simulink model "sim_1_twolink_joint_control_ideal"  (R2021a)
settings: Solver=ode15s  StartTime=0.0  StopTime=15  RelTol=1e-5  EnableMultiTasking=on
values from neighbouring files (symbols this model uses):
  b1 = 0.01    [sim_params.m]    (also in sim_params_force.m)
  b2 = 0.01    [sim_params.m]    (also in sim_params_force.m)
  D = [zeros(n); eye(n)]    [control_comparison_script.m]    (also in gen_twolink_ss.m = reshape([0.0,0.0,0.0,0.0,0.0,0.0,0.0,0.0],[4,2]))
  D_T_Q = D'*Q    [control_comparison_script.m]
  epsilon = 0.1    [control_comparison_script.m]
  g = 9.80665    [sim_params.m]    (also in sim_params_force.m)
  Kd1 = 2.5    [control_comparison_script.m]
  Kd1_grav = 2.5    [control_comparison_script.m]
  Kd1_inv = 12    [control_comparison_script.m]
  Kd1_robust = 7    [control_comparison_script.m]
  Kd2 = 0.5    [control_comparison_script.m]
  Kd2_grav = 0.5    [control_comparison_script.m]
  Kd2_inv = 15    [control_comparison_script.m]
  Kd2_robust = 35    [control_comparison_script.m]
  Klqr = lqr(A,B,Q,R)    [control_comparison_script.m]
  Kp1 = 30    [control_comparison_script.m]
  Kp1_grav = 15    [control_comparison_script.m]
  Kp1_inv = 25    [control_comparison_script.m]
  Kp1_robust = 25    [control_comparison_script.m]
  Kp2 = 7    [control_comparison_script.m]
  Kp2_grav = 3.5    [control_comparison_script.m]
  Kp2_inv = 50    [control_comparison_script.m]
  Kp2_robust = 45    [control_comparison_script.m]
  Kpp = place(A,B,p)    [control_comparison_script.m]
  L1x = 0.3    [sim_params.m]    (also in sim_params_force.m)
  L1y = 0.050    (= 0.05)    [sim_params.m]    (also in sim_params_force.m)
  L1z = 0.05    [sim_params.m]    (also in sim_params_force.m)
  L2x = 0.15    [sim_params.m]    (also in sim_params_force.m = 0.3)
  L2y = 0.05    [sim_params.m]    (also in sim_params_force.m)
  L2z = 0.05    [sim_params.m]    (also in sim_params_force.m)
  m1 = m1*1.25    [control_comparison_script.m]    (also in sim_params.m = 2.775; sim_params_force.m = 2.775)
  m2 = m2*1.25    [control_comparison_script.m]    (also in sim_params.m = 1.3875; sim_params_force.m = 2.775)
  N1 = 100    [control_comparison_script.m]
  N1_grav = 100    [control_comparison_script.m]
  N1_inv = 50    [control_comparison_script.m]
  N1_robust = 50    [control_comparison_script.m]
  N2 = 100    [control_comparison_script.m]
  N2_grav = 100    [control_comparison_script.m]
  N2_inv = 50    [control_comparison_script.m]
  N2_robust = 50    [control_comparison_script.m]
  rho = [1;1]    [control_comparison_script.m]
  theta1_0 = 0    [sim_params.m]    (also in sim_params_force.m = 1.57079632679)
  theta1_dot_0 = 0    [sim_params.m]    (also in sim_params_force.m)
  theta2_0 = 0    [sim_params.m]    (also in sim_params_force.m = -1.57079632679)
  theta2_dot_0 = 0    [sim_params.m]    (also in sim_params_force.m)
  Tsample = 0.001    [sim_params.m]    (also in sim_params_force.m)
undefined symbols (not defined in the file or in its folder): Kd, Ki, Kp, N, sigbuilder_block, X, Y, Z
libraries: pid_lib x12, sm_lib x11, nesl_utility x10, simulink_extras x8, spsFirstOrderFilterLib x4, dspmtrx3 x1
(part 1 of 3)
settings Model: Creator=bhorton  LastModifiedBy=Petronas-Tareq
settings SolverCC: ZeroCrossAlgorithm=Adaptive  AlgebraicLoopSolver=TrustRegion
settings DataIOCC: ReturnWorkspaceOutputs=off
settings OptimizationCC: LifeSpan=inf
settings DebuggingCC: SFUnexpectedBacktrackingDiag=warning  SFNoUnconditionalDefaultTransitionDiag=warning  SFExecutionAtInitializationDiag=none  SFMachineParentedDataDiag=warning  ArithmeticOperatorsInVariantConditions=warning
settings SFSimCC: SimUseLocalCustomCode=off  CustomCodeUndefinedFunction=UseInterfaceOnly
settings RTWCC: RTWUseLocalCustomCode=off
settings CodeAppCC: StateflowObjectComments=on
settings GRTTargetCC: TargetLangStandard=C89/C90 (ANSI)
settings ConfigComp: CovMetricSettings=dw  CovSaveCumulativeToWorkspaceVar=on  CovSaveSingleToWorkspaceVar=on  CovExternalEMLEnable=off
settings SimscapeCC: SimscapeNormalizeSystem=off  SimscapeLogType=all  SimscapeLogDataHistory=10000
settings ExplorerConfigSet: InternalSimMechanicsExplorerSettings="<ExplorerConfiguration><canonicalview>planar_xy</canonicalview><AnimationSetting><BasePlaybackSpeed>1.0</BasePlaybackSpeed><PlaybackSpeedFactor>4.0</PlaybackSpeedFactor></AnimationSetting><TilePanel><TileInfo><Tiles Columns=\"1\" Count=\"1\" Rows=\"1\"><Column Weight=\"1\"/><Row Weight=\"1\"/><Tile Height=\"1\" Width=\"1\" X=\"0\" Y=\"0\"/></Tiles></TileInfo><SceneInfo><SceneViewer><BGColor><R>0</R><G>0</G><B>0</B></BGColor><Camera><DoPerspective>off</DoPerspective><Position><X>0.0447898824465682299</X><Y>-0.016656403258507535</Y><Z>0.999999954328562035</Z></Position><Center><X>0.0447898824465682299</X><Y>-0.016656403258507535</Y><Z>-4.56714379648559543e-08</Z></Center><Up><X>0</X><Y>1</Y><Z>0</Z></Up><ViewLimDist>1</ViewLimDist><YLim>0.67213509984740738</YLim><XLim>1.22520332234454554</XLim></Camera></SceneViewer></SceneInfo></TilePanel><MechEditorPanel><Cameras/><GfxPanelCameraMap/><VideoCreator><PlaybackSpeedRatio>1</PlaybackSpeedRatio><FrameRate>30</FrameRate><VideoFormat>Motion JPEG AVI</VideoFormat><FrameSize>auto</FrameSize></VideoCreator></MechEditorPanel></ExplorerConfiguration>"

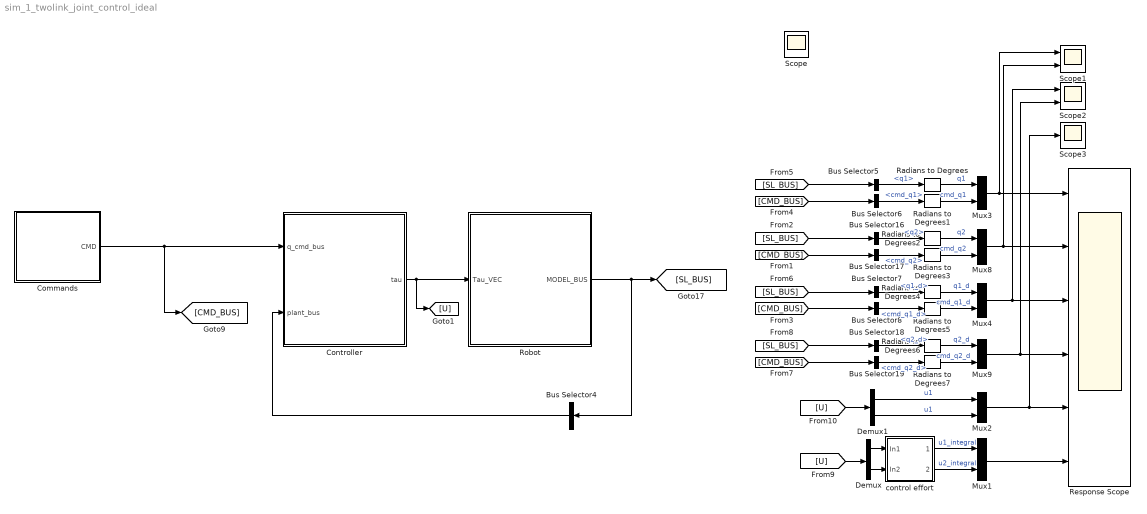
== system sim_1_twolink_joint_control_ideal ==
  Bus Selector16 : BusSelector  OutputSignals=q2
  Bus Selector17 : BusSelector  OutputSignals=cmd_q2
  Bus Selector18 : BusSelector  OutputSignals=q2_d
  Bus Selector19 : BusSelector  OutputSignals=cmd_q2_d
  Bus Selector4 : BusSelector  OutputSignals=q1_dd,q2_dd,q1_d,q2_d,q1,q2  OutputAsBus=on
  Bus Selector5 : BusSelector  OutputSignals=q1
  Bus Selector6 : BusSelector  OutputSignals=cmd_q1
  Bus Selector7 : BusSelector  OutputSignals=q1_d
  Bus Selector8 : BusSelector  OutputSignals=cmd_q1_d
  Commands : Subsystem  Variant=on  VariantControlMode=label  LabelModeActiveChoice=step
  Controller : Subsystem  Variant=on  VariantControlMode=label  LabelModeActiveChoice=LQR_control  PropagateVariantConditions=on
  Demux : Demux  Outputs=2
  Demux1 : Demux  Outputs=2
  Mux{1..4,8..9} (6 alike) : Mux  Inputs=2
  Radians to Degrees{,1..7} (8 alike) : simulink_extras/Transformations/Radians to Degrees
  Response Scope : Scope  NumInputPorts=6
  Robot : Subsystem  Variant=on  VariantControlMode=label  LabelModeActiveChoice=Choice
  Scope1 : Scope  NumInputPorts=2
  Scope2 : Scope  NumInputPorts=2
  Scope3 : Scope
  control effort : Subsystem
  Scope : Scope
  wires:
  Bus Selector4/1 -> Controller/2(plant_bus)
  Controller/1(tau) -> Robot/1(Tau_VEC), [U]
  Commands/1(CMD) -> [CMD_BUS], Controller/1(q_cmd_bus)
  Robot/1(MODEL_BUS) -> [SL_BUS], Bus Selector4/1
  Mux4/1 -> Scope2/1, Response Scope/3
  Mux8/1 -> Scope1/2, Response Scope/2
  Radians to Degrees4/1 -> Mux4/1  "q1_d"
  Radians to Degrees3/1 -> Mux8/2  "cmd_q2"
  Mux3/1 -> Scope1/1, Response Scope/1
  Radians to Degrees6/1 -> Mux9/1  "q2_d"
  Mux9/1 -> Scope2/2, Response Scope/4
  Radians to Degrees5/1 -> Mux4/2  "cmd_q1_d"
  Demux1/1 -> Mux2/1  "u1"
  [SL_BUS] -> Bus Selector7/1
  Bus Selector8/1 -> Radians to Degrees5/1  "<cmd_q1_d>"
  [CMD_BUS] -> Bus Selector8/1
  [U] -> Demux1/1
  Demux1/2 -> Mux2/2  "u1"
  control effort/2(u2_effort) -> Mux1/2  "u2_integral"
  Bus Selector16/1 -> Radians to Degrees2/1  "<q2>"
  [SL_BUS] -> Bus Selector5/1
  Demux/2 -> control effort/2(In2)
  control effort/1(u1_effort) -> Mux1/1  "u1_integral"
  Mux2/1 -> Scope3/1, Response Scope/5
  Bus Selector19/1 -> Radians to Degrees7/1  "<cmd_q2_d>"
  [CMD_BUS] -> Bus Selector19/1
  Bus Selector6/1 -> Radians to Degrees1/1  "<cmd_q1>"
  [SL_BUS] -> Bus Selector16/1
  Bus Selector17/1 -> Radians to Degrees3/1  "<cmd_q2>"
  [SL_BUS] -> Bus Selector18/1
  Radians to Degrees/1 -> Mux3/1  "q1"
  Radians to Degrees2/1 -> Mux8/1  "q2"
  Demux/1 -> control effort/1(In1)
  Bus Selector18/1 -> Radians to Degrees6/1  "<q2_d>"
  Bus Selector7/1 -> Radians to Degrees4/1  "<q1_d>"
  Bus Selector5/1 -> Radians to Degrees/1  "<q1>"
  Radians to Degrees1/1 -> Mux3/2  "cmd_q1"
  [U] -> Demux/1
  Mux1/1 -> Response Scope/6
  [CMD_BUS] -> Bus Selector17/1
  Radians to Degrees7/1 -> Mux9/2  "cmd_q2_d"
  [CMD_BUS] -> Bus Selector6/1

== system sim_1_twolink_joint_control_ideal/Commands ==
  Sinewave command : Subsystem  VariantControl=sinwave
  Step command : Subsystem  VariantControl=step
  Trapezoidal velocity : Subsystem  VariantControl=Trapezoidal velocity
  CMD : Outport

== system sim_1_twolink_joint_control_ideal/Controller ==
  note: 1) Add Subsystem or Model blocks as valid variant choices.
      | 2) You cannot connect blocks at this level. At simulation, connectivity is automatically
      | determined, based on the active variant and port name matching.
  q_cmd_bus : Inport
  plant_bus : Inport  Port=2
  "  LQR Control" : Subsystem  VariantControl=LQR_control
  " Pole Placement Control" : Subsystem  VariantControl=PolePlacement_control
  "Inverse Dynamics control " : Subsystem  VariantControl=Inverse_dynamics_control
  LQR+D Control : Subsystem  VariantControl=LQR_D_control
  PD Control : Subsystem  VariantControl=PD_control
  PD-feedforward-gravity Control : Subsystem  VariantControl=PD_plus_gravity_plus_feadforward
  "PD-gravity Control " : Subsystem  VariantControl=PD_plus_gravity
  PID Control : Subsystem  VariantControl=PID_control
  Pole Placement+D Control : Subsystem  VariantControl=PolePlacement_D_control
  "Robust control " : Subsystem  VariantControl=robust_control
  tau : Outport

== system sim_1_twolink_joint_control_ideal/Robot ==
  note: 1) Add Subsystem or Model blocks as valid variant choices.
      | 2) You cannot connect blocks at this level. At simulation, connectivity is automatically
      | determined, based on the active variant and port name matching.
  Tau_VEC : Inport
  SIMSCAPE_MODEL : Subsystem  VariantControl=Choice_1
  SIMULINK_MODEL : Subsystem  VariantControl=Choice
  MODEL_BUS : Outport

== system sim_1_twolink_joint_control_ideal/control effort ==
  In1 : Inport
  In2 : Inport  Port=2
  Integrator : Integrator
  Integrator1 : Integrator
  Square : Math  Operator=square  SaturateOnIntegerOverflow=on
  Square1 : Math  Operator=square  SaturateOnIntegerOverflow=on
  u1_effort : Outport
  u2_effort : Outport  Port=2
  wires:
  Square/1 -> Integrator/1
  Integrator1/1 -> u2_effort/1  "u2_effort"
  Integrator/1 -> u1_effort/1  "u1_effort"
  Square1/1 -> Integrator1/1
  In2/1 -> Square1/1
  In1/1 -> Square/1

== system sim_1_twolink_joint_control_ideal/Commands/Sinewave command ==
  note: Note: Using derivative blocks without limiters can result in spikes in the signal. Better to manually create the derivative of the signal
  Bus Creator : BusCreator  Inputs=6
  Derivative : Derivative
  Derivative1 : Derivative
  Gain : Gain  Gain=-1
  Gain1 : Gain  Gain=-1
  Sine Wave Function : Sin  SampleTime=0
  Sine Wave Function1 : Sin  Amplitude=0.5  SampleTime=0
  CMD : Outport
  wires:
  Bus Creator/1 -> CMD/1
  Sine Wave Function1/1 -> Gain1/1, Derivative1/1, Bus Creator/6  "cmd_q2"
  Gain1/1 -> Bus Creator/2  "cmd_q2_dd"
  Gain/1 -> Bus Creator/1  "cmd_q1_dd"
  Sine Wave Function/1 -> Gain/1, Derivative/1, Bus Creator/5  "cmd_q1"
  Derivative/1 -> Bus Creator/3  "cmd_q1_d"
  Derivative1/1 -> Bus Creator/4  "cmd_q2_d"

== system sim_1_twolink_joint_control_ideal/Commands/Step command ==
  Bus Creator : BusCreator  Inputs=6
  Constant : Constant  Value=0
  Constant1 : Constant  Value=0
  Derivative : Derivative
  Derivative1 : Derivative
  First-Order Filter : spsFirstOrderFilterLib/First-Order Filter  FilterType=Lowpass  Tc=0.3  Ts=0  Initialize=on  Vac_Init=[0, 0, 100]  Vdc_Init=0  PlotResponse=off  FreqRange="[0,  200,  1]"
  First-Order Filter1 : spsFirstOrderFilterLib/First-Order Filter  FilterType=Lowpass  Tc=0.3  Ts=0  Initialize=on  Vac_Init=[0, 0, 100]  Vdc_Init=0  PlotResponse=off  FreqRange="[0,  200,  1]"
  First-Order Filter2 : spsFirstOrderFilterLib/First-Order Filter  FilterType=Lowpass  Tc=0.2  Ts=0  Initialize=on  Vac_Init=[0, 0, 100]  Vdc_Init=0  PlotResponse=off  FreqRange="[0,  200,  1]"
  First-Order Filter3 : spsFirstOrderFilterLib/First-Order Filter  FilterType=Lowpass  Tc=0.2  Ts=0  Initialize=on  Vac_Init=[0, 0, 100]  Vdc_Init=0  PlotResponse=off  FreqRange="[0,  200,  1]"
  Joint commands : Subsystem  Tag=STV Subsys  LoadFcn=sigbuilder_block('load');  StartFcn=sigbuilder_block('start');  StopFcn=sigbuilder_block('stop');  ClipboardFcn=sigbuilder_block('clipboard');  mask(Sigbuilder block){tuvar=[0:10]}
      mask help: Simulink:masks:SigbuilderBlock_MD
      mask init:
      | if ~strcmp(get_param(bdroot(gcbh),'SimulationStatus'),'stopped') tuvar = sigbuilder_block('maskInit'); end
      settings: CopyFcn=sigbuilder_block('copy');  DeleteFcn=sigbuilder_block('delete');  ModelCloseFcn=sigbuilder_block('modelClose');  PreSaveFcn=sigbuilder_block('preSave');  PauseFcn=sigbuilder_block('pause');  ContinueFcn=sigbuilder_block('continue');  NameChangeFcn=sigbuilder_block('namechange');  OpenFcn=sigbuilder_block('open',[0 36 1152 560.4 ]);  CloseFcn=sigbuilder_block('close');
      mask Display: plot(0, 0, 100, 100,[2, 2, 32, 32, 2], [68, 8, 8, 68, 68],[32, 2], [38, 38], [32, 19, 2],[53, 60, 44], [32, 17, 17, 2],[16, 16, 31, 31]);txt = getActiveGroup(gcbh);text(2, 100, txt,'verticalAlignment', 'top');
  Scope : Scope
  Scope1 : Scope
  Zero-Order Hold : ZeroOrderHold  SampleTime=0.001
  CMD : Outport
  wires:
  Derivative1/1 -> First-Order Filter2/1
  First-Order Filter1/1 -> Bus Creator/5, Derivative/1  "cmd_q1"
  Bus Creator/1 -> Zero-Order Hold/1
  First-Order Filter/1 -> Derivative1/1, Bus Creator/6  "cmd_q2"
  Joint commands/2(cmd_q2) -> First-Order Filter/1  "cmd_q2"
  Derivative/1 -> Scope/1, First-Order Filter3/1
  Joint commands/1(cmd_q1) -> First-Order Filter1/1  "cmd_q1"
  Constant/1 -> Bus Creator/1  "cmd_q1_dd"
  Constant1/1 -> Bus Creator/2  "cmd_q2_dd"
  First-Order Filter2/1 -> Bus Creator/4  "cmd_q2_d"
  First-Order Filter3/1 -> Bus Creator/3  "cmd_q1_d"
  Zero-Order Hold/1 -> Scope1/1, CMD/1

== system sim_1_twolink_joint_control_ideal/Commands/Trapezoidal velocity ==
  Bus Creator : BusCreator  Inputs=6
  Derivative : Derivative
  Derivative2 : Derivative
  Integrator : Integrator
  Integrator1 : Integrator
  Joint commands : Subsystem  Tag=STV Subsys  LoadFcn=sigbuilder_block('load');  StartFcn=sigbuilder_block('start');  StopFcn=sigbuilder_block('stop');  ClipboardFcn=sigbuilder_block('clipboard');  mask(Sigbuilder block){tuvar=[0:10]}
      mask help: Simulink:masks:SigbuilderBlock_MD
      mask init:
      | if ~strcmp(get_param(bdroot(gcbh),'SimulationStatus'),'stopped') tuvar = sigbuilder_block('maskInit'); end
      settings: CopyFcn=sigbuilder_block('copy');  DeleteFcn=sigbuilder_block('delete');  ModelCloseFcn=sigbuilder_block('modelClose');  PreSaveFcn=sigbuilder_block('preSave');  PauseFcn=sigbuilder_block('pause');  ContinueFcn=sigbuilder_block('continue');  NameChangeFcn=sigbuilder_block('namechange');  OpenFcn=sigbuilder_block('open',[4.8 36 1142.4 525.6 ]);  CloseFcn=sigbuilder_block('close');
      mask Display: plot(0, 0, 100, 100,[2, 2, 32, 32, 2], [68, 8, 8, 68, 68],[32, 2], [38, 38], [32, 19, 2],[53, 60, 44], [32, 17, 17, 2],[16, 16, 31, 31]);txt = getActiveGroup(gcbh);text(2, 100, txt,'verticalAlignment', 'top');
  Mux : Mux  Inputs=2
  Scope : Scope
  CMD : Outport
  wires:
  Bus Creator/1 -> CMD/1
  Integrator/1 -> Mux/2, Bus Creator/6  "cmd_q2"
  Derivative2/1 -> Bus Creator/2  "cmd_q2_dd"
  Joint commands/1(cmd_q1_dot) -> Integrator1/1, Derivative/1, Bus Creator/3  "cmd_q1_d"
  Derivative/1 -> Bus Creator/1  "cmd_q1_dd"
  Joint commands/2(cmd_q2_dot) -> Integrator/1, Derivative2/1, Bus Creator/4  "cmd_q2_d"
  Integrator1/1 -> Mux/1, Bus Creator/5  "cmd_q1"
  Mux/1 -> Scope/1

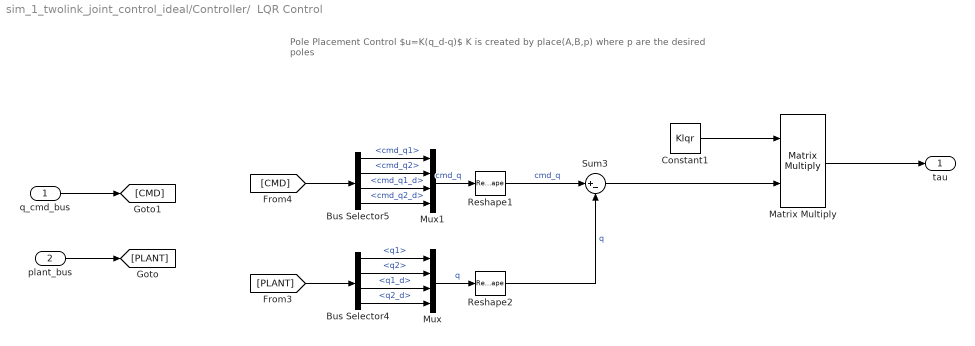
== system sim_1_twolink_joint_control_ideal/Controller/  LQR Control ==
  note: Pole Placement Control
      | $u=K(q_d-q)$
      | K is created by place(A,B,p) where p are the desired poles
  q_cmd_bus : Inport
  plant_bus : Inport  Port=2
  Bus Selector4 : BusSelector  OutputSignals=q1,q2,q1_d,q2_d
  Bus Selector5 : BusSelector  OutputSignals=cmd_q1,cmd_q2,cmd_q1_d,cmd_q2_d
  Constant1 : Constant  Value=Klqr  VectorParams1D=off
  Matrix Multiply : Product  Multiplication=Matrix(*)
  Mux : Mux
  Mux1 : Mux
  Reshape1 : Reshape  OutputDimensionality=Column vector (2-D)
  Reshape2 : Reshape  OutputDimensionality=Column vector (2-D)
  Sum3 : Sum  Inputs=|+-
  tau : Outport
  wires:
  plant_bus/1 -> [PLANT]
  q_cmd_bus/1 -> [CMD]
  [PLANT] -> Bus Selector4/1
  Bus Selector4/3 -> Mux/3  "<q1_d>"
  Bus Selector4/4 -> Mux/4  "<q2_d>"
  Mux/1 -> Reshape2/1  "q"
  Mux1/1 -> Reshape1/1  "cmd_q"
  [CMD] -> Bus Selector5/1
  Bus Selector5/3 -> Mux1/3  "<cmd_q1_d>"
  Bus Selector5/4 -> Mux1/4  "<cmd_q2_d>"
  Bus Selector5/2 -> Mux1/2  "<cmd_q2>"
  Bus Selector5/1 -> Mux1/1  "<cmd_q1>"
  Sum3/1 -> Matrix Multiply/2
  Reshape2/1 -> Sum3/2  "q"
  Reshape1/1 -> Sum3/1  "cmd_q"
  Constant1/1 -> Matrix Multiply/1
  Bus Selector4/1 -> Mux/1  "<q1>"
  Bus Selector4/2 -> Mux/2  "<q2>"
  Matrix Multiply/1 -> tau/1

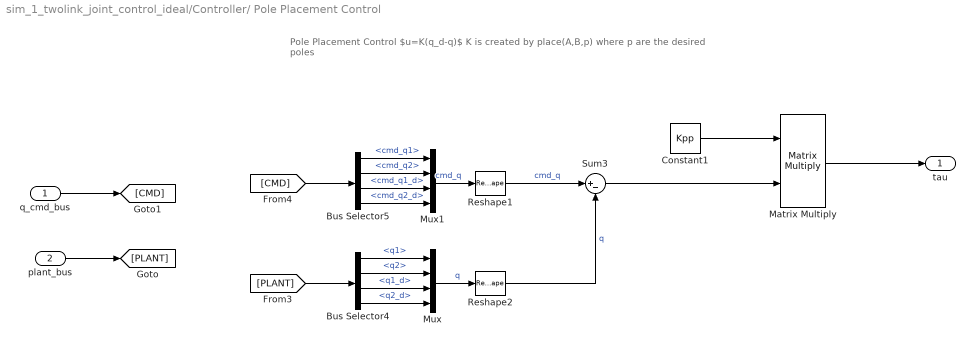
== system sim_1_twolink_joint_control_ideal/Controller/ Pole Placement Control ==
  note: Pole Placement Control
      | $u=K(q_d-q)$
      | K is created by place(A,B,p) where p are the desired poles
  q_cmd_bus : Inport
  plant_bus : Inport  Port=2
  Bus Selector4 : BusSelector  OutputSignals=q1,q2,q1_d,q2_d
  Bus Selector5 : BusSelector  OutputSignals=cmd_q1,cmd_q2,cmd_q1_d,cmd_q2_d
  Constant1 : Constant  Value=Kpp  VectorParams1D=off
  Matrix Multiply : Product  Multiplication=Matrix(*)
  Mux : Mux
  Mux1 : Mux
  Reshape1 : Reshape  OutputDimensionality=Column vector (2-D)
  Reshape2 : Reshape  OutputDimensionality=Column vector (2-D)
  Sum3 : Sum  Inputs=|+-
  tau : Outport
  wires:
  plant_bus/1 -> [PLANT]
  q_cmd_bus/1 -> [CMD]
  [PLANT] -> Bus Selector4/1
  Bus Selector4/3 -> Mux/3  "<q1_d>"
  Bus Selector4/4 -> Mux/4  "<q2_d>"
  Mux/1 -> Reshape2/1  "q"
  Mux1/1 -> Reshape1/1  "cmd_q"
  [CMD] -> Bus Selector5/1
  Bus Selector5/3 -> Mux1/3  "<cmd_q1_d>"
  Bus Selector5/4 -> Mux1/4  "<cmd_q2_d>"
  Bus Selector5/2 -> Mux1/2  "<cmd_q2>"
  Bus Selector5/1 -> Mux1/1  "<cmd_q1>"
  Sum3/1 -> Matrix Multiply/2
  Reshape2/1 -> Sum3/2  "q"
  Reshape1/1 -> Sum3/1  "cmd_q"
  Constant1/1 -> Matrix Multiply/1
  Bus Selector4/1 -> Mux/1  "<q1>"
  Bus Selector4/2 -> Mux/2  "<q2>"
  Matrix Multiply/1 -> tau/1

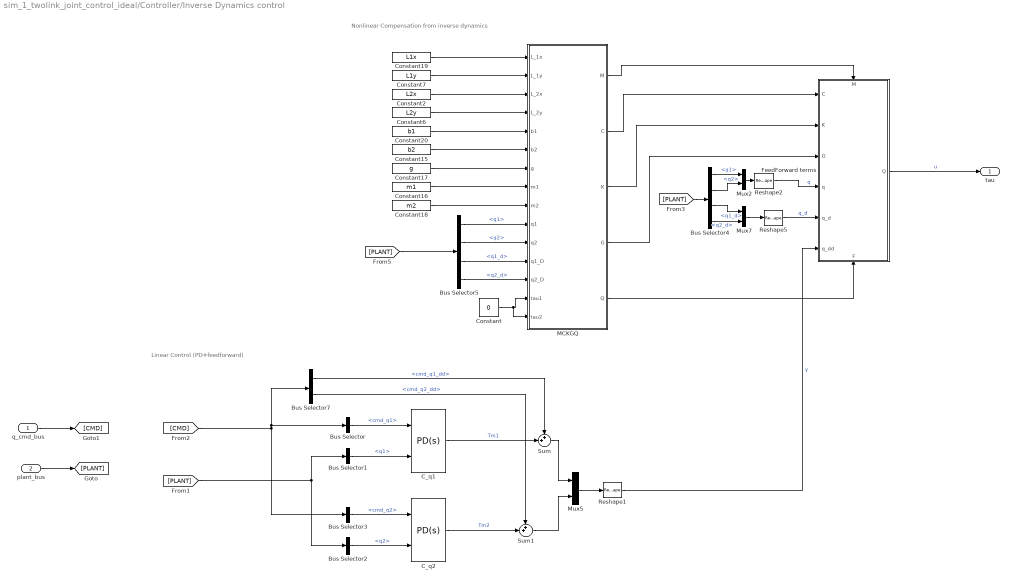
== system sim_1_twolink_joint_control_ideal/Controller/Inverse Dynamics control  ==
  note: Nonlinear Compensation from inverse dynamics
  note: Linear Control (PD+feedforward)
  q_cmd_bus : Inport
  plant_bus : Inport  Port=2
  Bus Selector : BusSelector  OutputSignals=cmd_q1
  Bus Selector1 : BusSelector  OutputSignals=q1
  Bus Selector2 : BusSelector  OutputSignals=q2
  Bus Selector3 : BusSelector  OutputSignals=cmd_q2
  Bus Selector4 : BusSelector  OutputSignals=q1,q2,q1_d,q2_d
  Bus Selector5 : BusSelector  OutputSignals=q1,q2,q1_d,q2_d
  Bus Selector7 : BusSelector  OutputSignals=cmd_q1_dd,cmd_q2_dd
  C_q1 : pid_lib/PID Controller (2DOF)  Controller=PD  Form=Parallel  TimeDomain=Continuous-time  UseExternalTs=off  SampleTime=-1  IntegratorMethod=Forward Euler  FilterMethod=Forward Euler  ControllerParametersSource=internal  P=Kp1_inv  I=20  D=Kd1_inv  UseFilter=on  N=N1_inv  b=1  c=1  TunerSelectOption=Transfer Function Based (PID Tuner App)  InitialConditionSource=internal  InitialConditionForIntegrator=0  InitialConditionForFilter=0  DifferentiatorICPrevScaledInput=0  ExternalReset=none  TrackingMode=off  Kt=1  LimitOutput=off  SatLimitsSource=internal  UpperSaturationLimit=inf  LowerSaturationLimit=-inf  LinearizeAsGain=on  AntiWindupMode=none  Kb=1  POutMin=[]  POutMax=[]  IOutMin=[]  IOutMax=[]  DOutMin=[]  DOutMax=[]  NOutMin=[]  NOutMax=[]  bOutMin=[]  bOutMax=[]  cOutMin=[]  cOutMax=[]  SumOutMin=[]  SumOutMax=[]  SaturationOutMin=[]  SaturationOutMax=[]  PParamMin=[]  PParamMax=[]  IParamMin=[]  IParamMax=[]  DParamMin=[]  DParamMax=[]  NParamMin=[]  NParamMax=[]  bParamMin=[]  bParamMax=[]  cParamMin=[]  cParamMax=[]  KbParamMin=[]  KbParamMax=[]  KtParamMin=[]  KtParamMax=[]  KbOutMin=[]  KbOutMax=[]  KtOutMin=[]  KtOutMax=[]  IntegratorOutMin=[]  IntegratorOutMax=[]  FilterOutMin=[]  FilterOutMax=[]  SumI1OutMin=[]  SumI1OutMax=[]  SumI2OutMin=[]  SumI2OutMax=[]  SumI3OutMin=[]  SumI3OutMax=[]  SumI4OutMin=[]  SumI4OutMax=[]  SumDOutMin=[]  SumDOutMax=[]  Sum1OutMin=[]  Sum1OutMax=[]  Sum2OutMin=[]  Sum2OutMax=[]  Sum3OutMin=[]  Sum3OutMax=[]  DifferentiatorOutMin=[]  DifferentiatorOutMax=[]  FilterDiffOutCoefMin=[]  FilterDiffOutCoefMax=[]  ReciprocalOutMin=[]  ReciprocalOutMax=[]  SumDenOutMin=[]  SumDenOutMax=[]  SumNumOutMin=[]  SumNumOutMax=[]  DivideOutMin=[]  DivideOutMax=[]  UdiffTsProdOutMin=[]  UdiffTsProdOutMax=[]  NTsProdOutMin=[]  NTsProdOutMax=[]  UintegralTsProdOutMin=[]  UintegralTsProdOutMax=[]  UngainTsProdOutMin=[]  UngainTsProdOutMax=[]  IntegratorContinuousStateAttributes=''  IntegratorStateMustResolveToSignalObject=off  IntegratorRTWStateStorageClass=Auto  FilterContinuousStateAttributes=''  FilterStateMustResolveToSignalObject=off  FilterRTWStateStorageClass=Auto  ParallelPVariant=InternalParameters  IdealPVariant=Disabled  IVariant=Disabled  DVariant=InternalParameters  bVariant=InternalParameters  cVariant=InternalParameters  IntegratorVariant=Disabled  SatVariant=Disabled  AWVariant=Disabled  PCopyVariant=Disabled  TRVariant=Disabled  FdbkBlocksVariant=Forward  IdealPFdbkVariant=Disabled  SatFdbkVariant=Disabled  DerivativeFilterVariant=ContFilter  NVariant=InternalParameters  NCopyVariant=Disabled  FilterICVariant=InternalICsFilter  IntegratorICVariant=Disabled  ExternalResetVariant=Disabled  TRSumVariant=Passthrough  SumFdbkVariant=Disabled  SumVariant=Sum_PD  TsampFilterVariant=InternalTs  TsampNgainVariant=Passthrough  TsampIntegralVariant=Disabled_SignalSpec  ExternalSaturationOutDataTypeStr=Inherit: Same as second input
      settings: SourceProductBaseCode=SL
  C_q2 : pid_lib/PID Controller (2DOF)  Controller=PD  Form=Parallel  TimeDomain=Continuous-time  UseExternalTs=off  SampleTime=-1  IntegratorMethod=Forward Euler  FilterMethod=Forward Euler  ControllerParametersSource=internal  P=Kp2_inv  I=20  D=Kd2_inv  UseFilter=on  N=N2_inv  b=1  c=1  TunerSelectOption=Transfer Function Based (PID Tuner App)  InitialConditionSource=internal  InitialConditionForIntegrator=0  InitialConditionForFilter=0  DifferentiatorICPrevScaledInput=0  ExternalReset=none  TrackingMode=off  Kt=1  LimitOutput=off  SatLimitsSource=internal  UpperSaturationLimit=inf  LowerSaturationLimit=-inf  LinearizeAsGain=on  AntiWindupMode=none  Kb=1  POutMin=[]  POutMax=[]  IOutMin=[]  IOutMax=[]  DOutMin=[]  DOutMax=[]  NOutMin=[]  NOutMax=[]  bOutMin=[]  bOutMax=[]  cOutMin=[]  cOutMax=[]  SumOutMin=[]  SumOutMax=[]  SaturationOutMin=[]  SaturationOutMax=[]  PParamMin=[]  PParamMax=[]  IParamMin=[]  IParamMax=[]  DParamMin=[]  DParamMax=[]  NParamMin=[]  NParamMax=[]  bParamMin=[]  bParamMax=[]  cParamMin=[]  cParamMax=[]  KbParamMin=[]  KbParamMax=[]  KtParamMin=[]  KtParamMax=[]  KbOutMin=[]  KbOutMax=[]  KtOutMin=[]  KtOutMax=[]  IntegratorOutMin=[]  IntegratorOutMax=[]  FilterOutMin=[]  FilterOutMax=[]  SumI1OutMin=[]  SumI1OutMax=[]  SumI2OutMin=[]  SumI2OutMax=[]  SumI3OutMin=[]  SumI3OutMax=[]  SumI4OutMin=[]  SumI4OutMax=[]  SumDOutMin=[]  SumDOutMax=[]  Sum1OutMin=[]  Sum1OutMax=[]  Sum2OutMin=[]  Sum2OutMax=[]  Sum3OutMin=[]  Sum3OutMax=[]  DifferentiatorOutMin=[]  DifferentiatorOutMax=[]  FilterDiffOutCoefMin=[]  FilterDiffOutCoefMax=[]  ReciprocalOutMin=[]  ReciprocalOutMax=[]  SumDenOutMin=[]  SumDenOutMax=[]  SumNumOutMin=[]  SumNumOutMax=[]  DivideOutMin=[]  DivideOutMax=[]  UdiffTsProdOutMin=[]  UdiffTsProdOutMax=[]  NTsProdOutMin=[]  NTsProdOutMax=[]  UintegralTsProdOutMin=[]  UintegralTsProdOutMax=[]  UngainTsProdOutMin=[]  UngainTsProdOutMax=[]  IntegratorContinuousStateAttributes=''  IntegratorStateMustResolveToSignalObject=off  IntegratorRTWStateStorageClass=Auto  FilterContinuousStateAttributes=''  FilterStateMustResolveToSignalObject=off  FilterRTWStateStorageClass=Auto  ParallelPVariant=InternalParameters  IdealPVariant=Disabled  IVariant=Disabled  DVariant=InternalParameters  bVariant=InternalParameters  cVariant=InternalParameters  IntegratorVariant=Disabled  SatVariant=Disabled  AWVariant=Disabled  PCopyVariant=Disabled  TRVariant=Disabled  FdbkBlocksVariant=Forward  IdealPFdbkVariant=Disabled  SatFdbkVariant=Disabled  DerivativeFilterVariant=ContFilter  NVariant=InternalParameters  NCopyVariant=Disabled  FilterICVariant=InternalICsFilter  IntegratorICVariant=Disabled  ExternalResetVariant=Disabled  TRSumVariant=Passthrough  SumFdbkVariant=Disabled  SumVariant=Sum_PD  TsampFilterVariant=InternalTs  TsampNgainVariant=Passthrough  TsampIntegralVariant=Disabled_SignalSpec  ExternalSaturationOutDataTypeStr=Inherit: Same as second input
      settings: SourceProductBaseCode=SL
  Constant : Constant  Value=0
  Constant15 : Constant  Value=b2
  Constant16 : Constant  Value=m1
  Constant17 : Constant  Value=g
  Constant18 : Constant  Value=m2
  Constant19 : Constant  Value=L1x
  Constant2 : Constant  Value=L2x
  Constant20 : Constant  Value=b1
  Constant6 : Constant  Value=L2y
  Constant7 : Constant  Value=L1y
  FeedForward terms : Subsystem
      settings: PortSchema="{\"entries\":[{\"content\":{\"sides\":[{\"content\":{\"connectorIds\":[\"In1\",\"In2\",\"In3\",\"In4\",\"In5\",\"In6\"]},\"type\":\"ConnectorPlacement.EquallySpacedRectSide\",\"uuid\":\"236e7a2f-027c-4887-b3e9-bc0e11a59ec6\"},{\"content\":{\"connectorIds\":[\"Out1\"],\"side\":\"RIGHT\"},\"type\":\"ConnectorPlacement.EquallySpacedRectSide\",\"uuid\":\"0b727d96-7650-4ea0-95ac-5fb1bad7af10\"},{\"content\":{\"connectorIds\":[\"In7\"],\"side\":\"TOP\"},\"type\":\"ConnectorPlacement.EquallySpacedRectSide\",\"uuid\":\"19d9c8c6-ae7e-49b4-b718-472bd3040569\"},{\"content\":{\"connectorIds\":[\"In8\"],\"side\":\"BOTTOM\"},\"type\":\"ConnectorPlacement.EquallySpacedRectSide\",\"uuid\":\"734f5953-872d-4718-8798-69ea98da43e1\"}]},\"type\":\"ConnectorPlacement.EquallySpacedConnector\",\"uuid\":\"f4b93fea-e2dd-47f1-bf2a-cf2dec03adb9\"}],\"packageUris\":[\"http://schema.mathworks.com/mf0/Connector/R2020b\"],\"version\":\"1.0\"}"
  MCKGQ : MATLAB Function  TreatAsAtomicUnit=on
  Mux2 : Mux  Inputs=2
  Mux5 : Mux  Inputs=2
  Mux7 : Mux  Inputs=2
  Reshape1 : Reshape  OutputDimensionality=Column vector (2-D)
  Reshape2 : Reshape  OutputDimensionality=Column vector (2-D)
  Reshape5 : Reshape  OutputDimensionality=Column vector (2-D)
  Sum : Sum  Inputs=++|
  Sum1 : Sum  Inputs=++|
  tau : Outport
  wires:
  C_q1/1 -> Sum/2  "Tm1"
  q_cmd_bus/1 -> [CMD]
  plant_bus/1 -> [PLANT]
  Bus Selector2/1 -> C_q2/2  "<q2>"
  Bus Selector3/1 -> C_q2/1  "<cmd_q2>"
  Bus Selector1/1 -> C_q1/2  "<q1>"
  Bus Selector/1 -> C_q1/1  "<cmd_q1>"
  [PLANT] -> Bus Selector1/1, Bus Selector2/1
  Bus Selector5/4 -> MCKGQ/13(q2_D)  "<q2_d>"
  Bus Selector5/3 -> MCKGQ/12(q1_D)  "<q1_d>"
  Bus Selector5/1 -> MCKGQ/10(q1)  "<q1>"
  [PLANT] -> Bus Selector5/1
  Bus Selector5/2 -> MCKGQ/11(q2)  "<q2>"
  Mux5/1 -> Reshape1/1
  FeedForward terms/1(Q) -> tau/1  "u"
  [CMD] -> Bus Selector7/1, Bus Selector/1, Bus Selector3/1
  Bus Selector7/2 -> Sum1/1  "<cmd_q2_dd>"
  Sum/1 -> Mux5/1
  C_q2/1 -> Sum1/2  "Tm2"
  Sum1/1 -> Mux5/2
  [PLANT] -> Bus Selector4/1
  Bus Selector4/3 -> Mux7/1  "<q1_d>"
  Bus Selector4/4 -> Mux7/2  "<q2_d>"
  Mux7/1 -> Reshape5/1
  Reshape5/1 -> FeedForward terms/5(q_d)  "q_d"
  Reshape1/1 -> FeedForward terms/6(q_dd)  "y"
  MCKGQ/2(C) -> FeedForward terms/1(C)
  MCKGQ/3(K) -> FeedForward terms/2(K)
  MCKGQ/4(G) -> FeedForward terms/3(G)
  Bus Selector4/1 -> Mux2/1  "<q1>"
  Bus Selector4/2 -> Mux2/2  "<q2>"
  Mux2/1 -> Reshape2/1
  Reshape2/1 -> FeedForward terms/4(q)  "q"
  Bus Selector7/1 -> Sum/1  "<cmd_q1_dd>"
  MCKGQ/5(Q) -> FeedForward terms/8(F)
  Constant/1 -> MCKGQ/14(tau1), MCKGQ/15(tau2)
  MCKGQ/1(M) -> FeedForward terms/7(M)
  Constant7/1 -> MCKGQ/2(L_1y)
  Constant2/1 -> MCKGQ/3(L_2x)
  Constant6/1 -> MCKGQ/4(L_2y)
  Constant20/1 -> MCKGQ/5(b1)
  Constant15/1 -> MCKGQ/6(b2)
  Constant17/1 -> MCKGQ/7(g)
  Constant16/1 -> MCKGQ/8(m1)
  Constant18/1 -> MCKGQ/9(m2)
  Constant19/1 -> MCKGQ/1(L_1x)

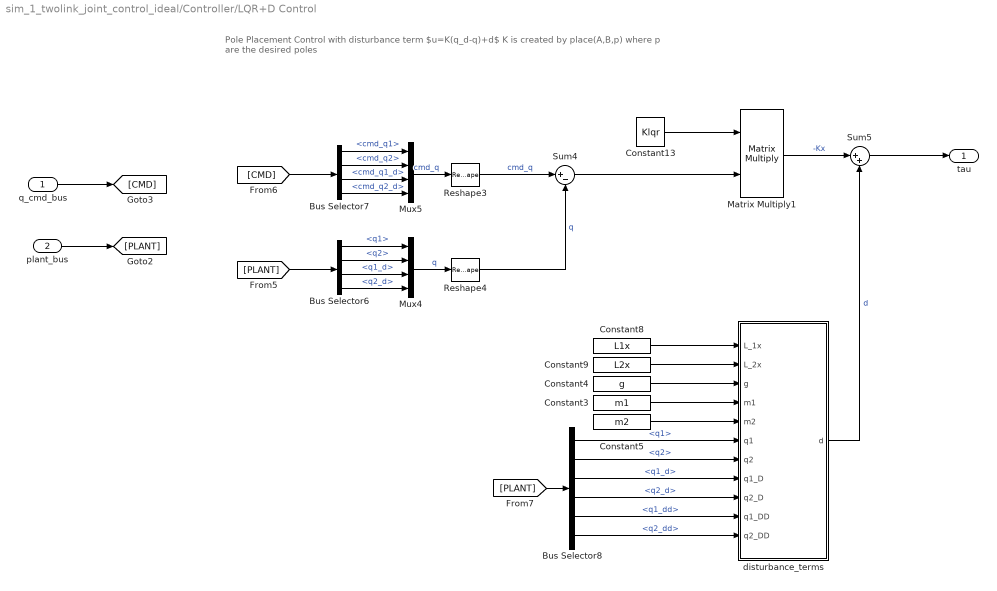
== system sim_1_twolink_joint_control_ideal/Controller/LQR+D Control ==
  note: Pole Placement Control with disturbance term
      | $u=K(q_d-q)+d$
      | K is created by place(A,B,p) where p are the desired poles
  q_cmd_bus : Inport
  plant_bus : Inport  Port=2
  Bus Selector6 : BusSelector  OutputSignals=q1,q2,q1_d,q2_d
  Bus Selector7 : BusSelector  OutputSignals=cmd_q1,cmd_q2,cmd_q1_d,cmd_q2_d
  Bus Selector8 : BusSelector  OutputSignals=q1,q2,q1_d,q2_d,q1_dd,q2_dd
  Constant13 : Constant  Value=Klqr  VectorParams1D=off
  Constant3 : Constant  Value=m1
  Constant4 : Constant  Value=g
  Constant5 : Constant  Value=m2
  Constant8 : Constant  Value=L1x
  Constant9 : Constant  Value=L2x
  Matrix Multiply1 : Product  Multiplication=Matrix(*)
  Mux4 : Mux
  Mux5 : Mux
  Reshape3 : Reshape  OutputDimensionality=Column vector (2-D)
  Reshape4 : Reshape  OutputDimensionality=Column vector (2-D)
  Sum4 : Sum  Inputs=|+-
  Sum5 : Sum  Inputs=|++
  disturbance_terms : MATLAB Function  TreatAsAtomicUnit=on
  tau : Outport
  wires:
  Bus Selector6/2 -> Mux4/2  "<q2>"
  Bus Selector6/1 -> Mux4/1  "<q1>"
  Mux4/1 -> Reshape4/1  "q"
  q_cmd_bus/1 -> [CMD]
  plant_bus/1 -> [PLANT]
  Mux5/1 -> Reshape3/1  "cmd_q"
  Bus Selector6/3 -> Mux4/3  "<q1_d>"
  [PLANT] -> Bus Selector6/1
  Bus Selector6/4 -> Mux4/4  "<q2_d>"
  Reshape3/1 -> Sum4/1  "cmd_q"
  Reshape4/1 -> Sum4/2  "q"
  Matrix Multiply1/1 -> Sum5/1  "-Kx"
  Sum4/1 -> Matrix Multiply1/2
  Bus Selector7/1 -> Mux5/1  "<cmd_q1>"
  Bus Selector7/2 -> Mux5/2  "<cmd_q2>"
  Bus Selector7/3 -> Mux5/3  "<cmd_q1_d>"
  Constant13/1 -> Matrix Multiply1/1
  Bus Selector7/4 -> Mux5/4  "<cmd_q2_d>"
  [CMD] -> Bus Selector7/1
  Sum5/1 -> tau/1
  disturbance_terms/1(d) -> Sum5/2  "d"
  [PLANT] -> Bus Selector8/1
  Bus Selector8/1 -> disturbance_terms/6(q1)  "<q1>"
  Bus Selector8/2 -> disturbance_terms/7(q2)  "<q2>"
  Bus Selector8/3 -> disturbance_terms/8(q1_D)  "<q1_d>"
  Bus Selector8/4 -> disturbance_terms/9(q2_D)  "<q2_d>"
  Bus Selector8/5 -> disturbance_terms/10(q1_DD)  "<q1_dd>"
  Bus Selector8/6 -> disturbance_terms/11(q2_DD)  "<q2_dd>"
  Constant8/1 -> disturbance_terms/1(L_1x)
  Constant9/1 -> disturbance_terms/2(L_2x)
  Constant4/1 -> disturbance_terms/3(g)
  Constant3/1 -> disturbance_terms/4(m1)
  Constant5/1 -> disturbance_terms/5(m2)

== system sim_1_twolink_joint_control_ideal/Controller/PD Control ==
  note: PD Joint Control
  q_cmd_bus : Inport
  plant_bus : Inport  Port=2
  Bus Selector : BusSelector  OutputSignals=cmd_q1
  Bus Selector1 : BusSelector  OutputSignals=q1
  Bus Selector2 : BusSelector  OutputSignals=q2
  Bus Selector3 : BusSelector  OutputSignals=cmd_q2
  C_q1 : pid_lib/PID Controller (2DOF)  Controller=PD  Form=Parallel  TimeDomain=Continuous-time  UseExternalTs=off  SampleTime=-1  IntegratorMethod=Forward Euler  FilterMethod=Forward Euler  ControllerParametersSource=internal  P=Kp1  I=20  D=Kd1  UseFilter=on  N=N1  b=1  c=1  TunerSelectOption=Transfer Function Based (PID Tuner App)  InitialConditionSource=internal  InitialConditionForIntegrator=0  InitialConditionForFilter=0  DifferentiatorICPrevScaledInput=0  ExternalReset=none  TrackingMode=off  Kt=1  LimitOutput=off  SatLimitsSource=internal  UpperSaturationLimit=inf  LowerSaturationLimit=-inf  LinearizeAsGain=on  AntiWindupMode=none  Kb=1  POutMin=[]  POutMax=[]  IOutMin=[]  IOutMax=[]  DOutMin=[]  DOutMax=[]  NOutMin=[]  NOutMax=[]  bOutMin=[]  bOutMax=[]  cOutMin=[]  cOutMax=[]  SumOutMin=[]  SumOutMax=[]  SaturationOutMin=[]  SaturationOutMax=[]  PParamMin=[]  PParamMax=[]  IParamMin=[]  IParamMax=[]  DParamMin=[]  DParamMax=[]  NParamMin=[]  NParamMax=[]  bParamMin=[]  bParamMax=[]  cParamMin=[]  cParamMax=[]  KbParamMin=[]  KbParamMax=[]  KtParamMin=[]  KtParamMax=[]  KbOutMin=[]  KbOutMax=[]  KtOutMin=[]  KtOutMax=[]  IntegratorOutMin=[]  IntegratorOutMax=[]  FilterOutMin=[]  FilterOutMax=[]  SumI1OutMin=[]  SumI1OutMax=[]  SumI2OutMin=[]  SumI2OutMax=[]  SumI3OutMin=[]  SumI3OutMax=[]  SumI4OutMin=[]  SumI4OutMax=[]  SumDOutMin=[]  SumDOutMax=[]  Sum1OutMin=[]  Sum1OutMax=[]  Sum2OutMin=[]  Sum2OutMax=[]  Sum3OutMin=[]  Sum3OutMax=[]  DifferentiatorOutMin=[]  DifferentiatorOutMax=[]  FilterDiffOutCoefMin=[]  FilterDiffOutCoefMax=[]  ReciprocalOutMin=[]  ReciprocalOutMax=[]  SumDenOutMin=[]  SumDenOutMax=[]  SumNumOutMin=[]  SumNumOutMax=[]  DivideOutMin=[]  DivideOutMax=[]  UdiffTsProdOutMin=[]  UdiffTsProdOutMax=[]  NTsProdOutMin=[]  NTsProdOutMax=[]  UintegralTsProdOutMin=[]  UintegralTsProdOutMax=[]  UngainTsProdOutMin=[]  UngainTsProdOutMax=[]  IntegratorContinuousStateAttributes=''  IntegratorStateMustResolveToSignalObject=off  IntegratorRTWStateStorageClass=Auto  FilterContinuousStateAttributes=''  FilterStateMustResolveToSignalObject=off  FilterRTWStateStorageClass=Auto  ParallelPVariant=InternalParameters  IdealPVariant=Disabled  IVariant=Disabled  DVariant=InternalParameters  bVariant=InternalParameters  cVariant=InternalParameters  IntegratorVariant=Disabled  SatVariant=Disabled  AWVariant=Disabled  PCopyVariant=Disabled  TRVariant=Disabled  FdbkBlocksVariant=Forward  IdealPFdbkVariant=Disabled  SatFdbkVariant=Disabled  DerivativeFilterVariant=ContFilter  NVariant=InternalParameters  NCopyVariant=Disabled  FilterICVariant=InternalICsFilter  IntegratorICVariant=Disabled  ExternalResetVariant=Disabled  TRSumVariant=Passthrough  SumFdbkVariant=Disabled  SumVariant=Sum_PD  TsampFilterVariant=InternalTs  TsampNgainVariant=Passthrough  TsampIntegralVariant=Disabled_SignalSpec  ExternalSaturationOutDataTypeStr=Inherit: Same as second input
      settings: SourceProductBaseCode=SL
  C_q2 : pid_lib/PID Controller (2DOF)  Controller=PD  Form=Parallel  TimeDomain=Continuous-time  UseExternalTs=off  SampleTime=-1  IntegratorMethod=Forward Euler  FilterMethod=Forward Euler  ControllerParametersSource=internal  P=Kp2  I=307.702571204868  D=Kd2  UseFilter=on  N=N2  b=1  c=1  TunerSelectOption=Transfer Function Based (PID Tuner App)  InitialConditionSource=internal  InitialConditionForIntegrator=0  InitialConditionForFilter=0  DifferentiatorICPrevScaledInput=0  ExternalReset=none  TrackingMode=off  Kt=1  LimitOutput=off  SatLimitsSource=internal  UpperSaturationLimit=inf  LowerSaturationLimit=-inf  LinearizeAsGain=on  AntiWindupMode=none  Kb=1  POutMin=[]  POutMax=[]  IOutMin=[]  IOutMax=[]  DOutMin=[]  DOutMax=[]  NOutMin=[]  NOutMax=[]  bOutMin=[]  bOutMax=[]  cOutMin=[]  cOutMax=[]  SumOutMin=[]  SumOutMax=[]  SaturationOutMin=[]  SaturationOutMax=[]  PParamMin=[]  PParamMax=[]  IParamMin=[]  IParamMax=[]  DParamMin=[]  DParamMax=[]  NParamMin=[]  NParamMax=[]  bParamMin=[]  bParamMax=[]  cParamMin=[]  cParamMax=[]  KbParamMin=[]  KbParamMax=[]  KtParamMin=[]  KtParamMax=[]  KbOutMin=[]  KbOutMax=[]  KtOutMin=[]  KtOutMax=[]  IntegratorOutMin=[]  IntegratorOutMax=[]  FilterOutMin=[]  FilterOutMax=[]  SumI1OutMin=[]  SumI1OutMax=[]  SumI2OutMin=[]  SumI2OutMax=[]  SumI3OutMin=[]  SumI3OutMax=[]  SumI4OutMin=[]  SumI4OutMax=[]  SumDOutMin=[]  SumDOutMax=[]  Sum1OutMin=[]  Sum1OutMax=[]  Sum2OutMin=[]  Sum2OutMax=[]  Sum3OutMin=[]  Sum3OutMax=[]  DifferentiatorOutMin=[]  DifferentiatorOutMax=[]  FilterDiffOutCoefMin=[]  FilterDiffOutCoefMax=[]  ReciprocalOutMin=[]  ReciprocalOutMax=[]  SumDenOutMin=[]  SumDenOutMax=[]  SumNumOutMin=[]  SumNumOutMax=[]  DivideOutMin=[]  DivideOutMax=[]  UdiffTsProdOutMin=[]  UdiffTsProdOutMax=[]  NTsProdOutMin=[]  NTsProdOutMax=[]  UintegralTsProdOutMin=[]  UintegralTsProdOutMax=[]  UngainTsProdOutMin=[]  UngainTsProdOutMax=[]  IntegratorContinuousStateAttributes=''  IntegratorStateMustResolveToSignalObject=off  IntegratorRTWStateStorageClass=Auto  FilterContinuousStateAttributes=''  FilterStateMustResolveToSignalObject=off  FilterRTWStateStorageClass=Auto  ParallelPVariant=InternalParameters  IdealPVariant=Disabled  IVariant=Disabled  DVariant=InternalParameters  bVariant=InternalParameters  cVariant=InternalParameters  IntegratorVariant=Disabled  SatVariant=Disabled  AWVariant=Disabled  PCopyVariant=Disabled  TRVariant=Disabled  FdbkBlocksVariant=Forward  IdealPFdbkVariant=Disabled  SatFdbkVariant=Disabled  DerivativeFilterVariant=ContFilter  NVariant=InternalParameters  NCopyVariant=Disabled  FilterICVariant=InternalICsFilter  IntegratorICVariant=Disabled  ExternalResetVariant=Disabled  TRSumVariant=Passthrough  SumFdbkVariant=Disabled  SumVariant=Sum_PD  TsampFilterVariant=InternalTs  TsampNgainVariant=Passthrough  TsampIntegralVariant=Disabled_SignalSpec  ExternalSaturationOutDataTypeStr=Inherit: Same as second input
      settings: SourceProductBaseCode=SL
  Mux2 : Mux  Inputs=2
  tau : Outport
  wires:
  [CMD] -> Bus Selector3/1, Bus Selector/1
  [PLANT] -> Bus Selector2/1, Bus Selector1/1
  Bus Selector/1 -> C_q1/1  "<cmd_q1>"
  Bus Selector1/1 -> C_q1/2  "<q1>"
  Bus Selector3/1 -> C_q2/1  "<cmd_q2>"
  Bus Selector2/1 -> C_q2/2  "<q2>"
  plant_bus/1 -> [PLANT]
  q_cmd_bus/1 -> [CMD]
  C_q2/1 -> Mux2/2
  C_q1/1 -> Mux2/1
  Mux2/1 -> tau/1

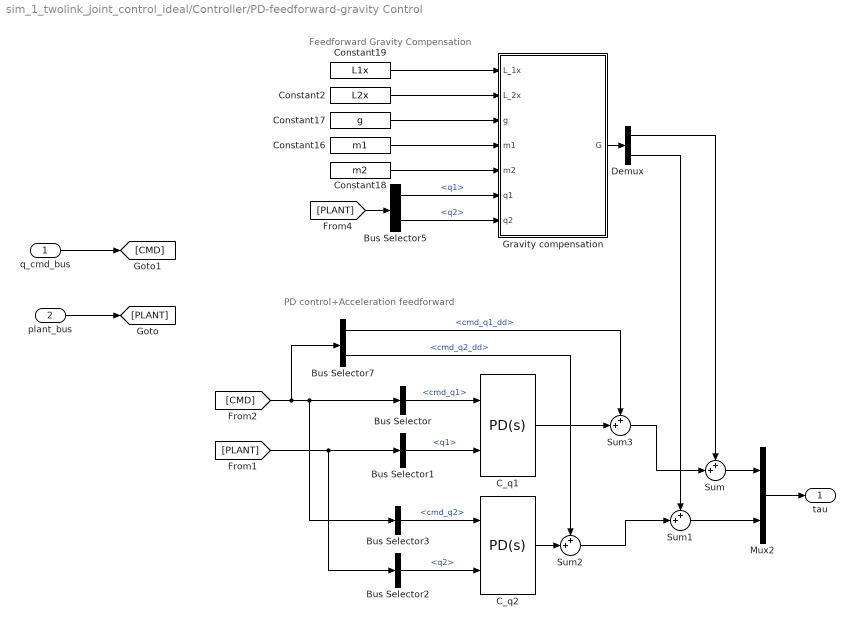
== system sim_1_twolink_joint_control_ideal/Controller/PD-feedforward-gravity Control ==
  note: PD control+Acceleration feedforward
  note: Feedforward Gravity Compensation
  q_cmd_bus : Inport
  plant_bus : Inport  Port=2
  Bus Selector : BusSelector  OutputSignals=cmd_q1
  Bus Selector1 : BusSelector  OutputSignals=q1
  Bus Selector2 : BusSelector  OutputSignals=q2
  Bus Selector3 : BusSelector  OutputSignals=cmd_q2
  Bus Selector5 : BusSelector  OutputSignals=q1,q2
  Bus Selector7 : BusSelector  OutputSignals=cmd_q1_dd,cmd_q2_dd
  C_q1 : pid_lib/PID Controller (2DOF)  Controller=PD  Form=Parallel  TimeDomain=Continuous-time  UseExternalTs=off  SampleTime=-1  IntegratorMethod=Forward Euler  FilterMethod=Forward Euler  ControllerParametersSource=internal  P=Kp1_grav  I=20  D=Kd1_grav  UseFilter=on  N=N1_grav  b=1  c=1  TunerSelectOption=Transfer Function Based (PID Tuner App)  InitialConditionSource=internal  InitialConditionForIntegrator=0  InitialConditionForFilter=0  DifferentiatorICPrevScaledInput=0  ExternalReset=none  TrackingMode=off  Kt=1  LimitOutput=off  SatLimitsSource=internal  UpperSaturationLimit=inf  LowerSaturationLimit=-inf  LinearizeAsGain=on  AntiWindupMode=none  Kb=1  POutMin=[]  POutMax=[]  IOutMin=[]  IOutMax=[]  DOutMin=[]  DOutMax=[]  NOutMin=[]  NOutMax=[]  bOutMin=[]  bOutMax=[]  cOutMin=[]  cOutMax=[]  SumOutMin=[]  SumOutMax=[]  SaturationOutMin=[]  SaturationOutMax=[]  PParamMin=[]  PParamMax=[]  IParamMin=[]  IParamMax=[]  DParamMin=[]  DParamMax=[]  NParamMin=[]  NParamMax=[]  bParamMin=[]  bParamMax=[]  cParamMin=[]  cParamMax=[]  KbParamMin=[]  KbParamMax=[]  KtParamMin=[]  KtParamMax=[]  KbOutMin=[]  KbOutMax=[]  KtOutMin=[]  KtOutMax=[]  IntegratorOutMin=[]  IntegratorOutMax=[]  FilterOutMin=[]  FilterOutMax=[]  SumI1OutMin=[]  SumI1OutMax=[]  SumI2OutMin=[]  SumI2OutMax=[]  SumI3OutMin=[]  SumI3OutMax=[]  SumI4OutMin=[]  SumI4OutMax=[]  SumDOutMin=[]  SumDOutMax=[]  Sum1OutMin=[]  Sum1OutMax=[]  Sum2OutMin=[]  Sum2OutMax=[]  Sum3OutMin=[]  Sum3OutMax=[]  DifferentiatorOutMin=[]  DifferentiatorOutMax=[]  FilterDiffOutCoefMin=[]  FilterDiffOutCoefMax=[]  ReciprocalOutMin=[]  ReciprocalOutMax=[]  SumDenOutMin=[]  SumDenOutMax=[]  SumNumOutMin=[]  SumNumOutMax=[]  DivideOutMin=[]  DivideOutMax=[]  UdiffTsProdOutMin=[]  UdiffTsProdOutMax=[]  NTsProdOutMin=[]  NTsProdOutMax=[]  UintegralTsProdOutMin=[]  UintegralTsProdOutMax=[]  UngainTsProdOutMin=[]  UngainTsProdOutMax=[]  IntegratorContinuousStateAttributes=''  IntegratorStateMustResolveToSignalObject=off  IntegratorRTWStateStorageClass=Auto  FilterContinuousStateAttributes=''  FilterStateMustResolveToSignalObject=off  FilterRTWStateStorageClass=Auto  ParallelPVariant=InternalParameters  IdealPVariant=Disabled  IVariant=Disabled  DVariant=InternalParameters  bVariant=InternalParameters  cVariant=InternalParameters  IntegratorVariant=Disabled  SatVariant=Disabled  AWVariant=Disabled  PCopyVariant=Disabled  TRVariant=Disabled  FdbkBlocksVariant=Forward  IdealPFdbkVariant=Disabled  SatFdbkVariant=Disabled  DerivativeFilterVariant=ContFilter  NVariant=InternalParameters  NCopyVariant=Disabled  FilterICVariant=InternalICsFilter  IntegratorICVariant=Disabled  ExternalResetVariant=Disabled  TRSumVariant=Passthrough  SumFdbkVariant=Disabled  SumVariant=Sum_PD  TsampFilterVariant=InternalTs  TsampNgainVariant=Passthrough  TsampIntegralVariant=Disabled_SignalSpec  ExternalSaturationOutDataTypeStr=Inherit: Same as second input
      settings: SourceProductBaseCode=SL
  C_q2 : pid_lib/PID Controller (2DOF)  Controller=PD  Form=Parallel  TimeDomain=Continuous-time  UseExternalTs=off  SampleTime=-1  IntegratorMethod=Forward Euler  FilterMethod=Forward Euler  ControllerParametersSource=internal  P=Kp2_grav  I=307.702571204868  D=Kd2_grav  UseFilter=on  N=N2_grav  b=1  c=1  TunerSelectOption=Transfer Function Based (PID Tuner App)  InitialConditionSource=internal  InitialConditionForIntegrator=0  InitialConditionForFilter=0  DifferentiatorICPrevScaledInput=0  ExternalReset=none  TrackingMode=off  Kt=1  LimitOutput=off  SatLimitsSource=internal  UpperSaturationLimit=inf  LowerSaturationLimit=-inf  LinearizeAsGain=on  AntiWindupMode=none  Kb=1  POutMin=[]  POutMax=[]  IOutMin=[]  IOutMax=[]  DOutMin=[]  DOutMax=[]  NOutMin=[]  NOutMax=[]  bOutMin=[]  bOutMax=[]  cOutMin=[]  cOutMax=[]  SumOutMin=[]  SumOutMax=[]  SaturationOutMin=[]  SaturationOutMax=[]  PParamMin=[]  PParamMax=[]  IParamMin=[]  IParamMax=[]  DParamMin=[]  DParamMax=[]  NParamMin=[]  NParamMax=[]  bParamMin=[]  bParamMax=[]  cParamMin=[]  cParamMax=[]  KbParamMin=[]  KbParamMax=[]  KtParamMin=[]  KtParamMax=[]  KbOutMin=[]  KbOutMax=[]  KtOutMin=[]  KtOutMax=[]  IntegratorOutMin=[]  IntegratorOutMax=[]  FilterOutMin=[]  FilterOutMax=[]  SumI1OutMin=[]  SumI1OutMax=[]  SumI2OutMin=[]  SumI2OutMax=[]  SumI3OutMin=[]  SumI3OutMax=[]  SumI4OutMin=[]  SumI4OutMax=[]  SumDOutMin=[]  SumDOutMax=[]  Sum1OutMin=[]  Sum1OutMax=[]  Sum2OutMin=[]  Sum2OutMax=[]  Sum3OutMin=[]  Sum3OutMax=[]  DifferentiatorOutMin=[]  DifferentiatorOutMax=[]  FilterDiffOutCoefMin=[]  FilterDiffOutCoefMax=[]  ReciprocalOutMin=[]  ReciprocalOutMax=[]  SumDenOutMin=[]  SumDenOutMax=[]  SumNumOutMin=[]  SumNumOutMax=[]  DivideOutMin=[]  DivideOutMax=[]  UdiffTsProdOutMin=[]  UdiffTsProdOutMax=[]  NTsProdOutMin=[]  NTsProdOutMax=[]  UintegralTsProdOutMin=[]  UintegralTsProdOutMax=[]  UngainTsProdOutMin=[]  UngainTsProdOutMax=[]  IntegratorContinuousStateAttributes=''  IntegratorStateMustResolveToSignalObject=off  IntegratorRTWStateStorageClass=Auto  FilterContinuousStateAttributes=''  FilterStateMustResolveToSignalObject=off  FilterRTWStateStorageClass=Auto  ParallelPVariant=InternalParameters  IdealPVariant=Disabled  IVariant=Disabled  DVariant=InternalParameters  bVariant=InternalParameters  cVariant=InternalParameters  IntegratorVariant=Disabled  SatVariant=Disabled  AWVariant=Disabled  PCopyVariant=Disabled  TRVariant=Disabled  FdbkBlocksVariant=Forward  IdealPFdbkVariant=Disabled  SatFdbkVariant=Disabled  DerivativeFilterVariant=ContFilter  NVariant=InternalParameters  NCopyVariant=Disabled  FilterICVariant=InternalICsFilter  IntegratorICVariant=Disabled  ExternalResetVariant=Disabled  TRSumVariant=Passthrough  SumFdbkVariant=Disabled  SumVariant=Sum_PD  TsampFilterVariant=InternalTs  TsampNgainVariant=Passthrough  TsampIntegralVariant=Disabled_SignalSpec  ExternalSaturationOutDataTypeStr=Inherit: Same as second input
      settings: SourceProductBaseCode=SL
  Constant16 : Constant  Value=m1
  Constant17 : Constant  Value=g
  Constant18 : Constant  Value=m2
  Constant19 : Constant  Value=L1x
  Constant2 : Constant  Value=L2x
  Demux : Demux  Outputs=2
  Gravity compensation : MATLAB Function  TreatAsAtomicUnit=on
  Mux2 : Mux  Inputs=2
  Sum{,1..3} (4 alike) : Sum  Inputs=++|
  tau : Outport
  wires:
  Mux2/1 -> tau/1
  Sum/1 -> Mux2/1
  Sum1/1 -> Mux2/2
  q_cmd_bus/1 -> [CMD]
  plant_bus/1 -> [PLANT]
  Demux/1 -> Sum/1
  Demux/2 -> Sum1/1
  C_q2/1 -> Sum2/2
  [CMD] -> Bus Selector7/1, Bus Selector3/1, Bus Selector/1
  [PLANT] -> Bus Selector2/1, Bus Selector1/1
  Bus Selector1/1 -> C_q1/2  "<q1>"
  Bus Selector2/1 -> C_q2/2  "<q2>"
  Bus Selector3/1 -> C_q2/1  "<cmd_q2>"
  Bus Selector/1 -> C_q1/1  "<cmd_q1>"
  C_q1/1 -> Sum3/2
  Sum3/1 -> Sum/2
  Sum2/1 -> Sum1/2
  Bus Selector7/1 -> Sum3/1  "<cmd_q1_dd>"
  Bus Selector7/2 -> Sum2/1  "<cmd_q2_dd>"
  Constant17/1 -> Gravity compensation/3(g)
  Constant18/1 -> Gravity compensation/5(m2)
  Bus Selector5/2 -> Gravity compensation/7(q2)  "<q2>"
  [PLANT] -> Bus Selector5/1
  Gravity compensation/1(G) -> Demux/1
  Constant19/1 -> Gravity compensation/1(L_1x)
  Constant2/1 -> Gravity compensation/2(L_2x)
  Bus Selector5/1 -> Gravity compensation/6(q1)  "<q1>"
  Constant16/1 -> Gravity compensation/4(m1)
